simulink model "IEEE9_SG_GFOR_GFOL"  (R2023b)
settings: Solver=ode1  StartTime=0.0  StopTime=sim_config.Tsim  RelTol=1e-3
undefined symbols (not defined in the file): sim_config
libraries: myLibrary x24, spsThreePhaseVIMeasurementLib x12, spsPower3phInstantaneousLib x6, spspowerguiLib x1
settings Model: Creator=Josep  LastModifiedBy=Josep

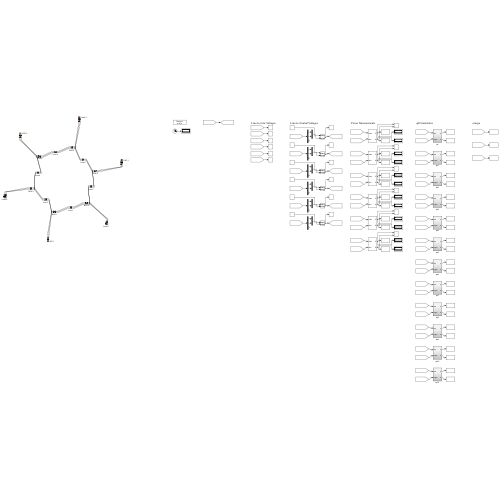
[thumbnail: Simulink's stored preview of the top-level diagram]
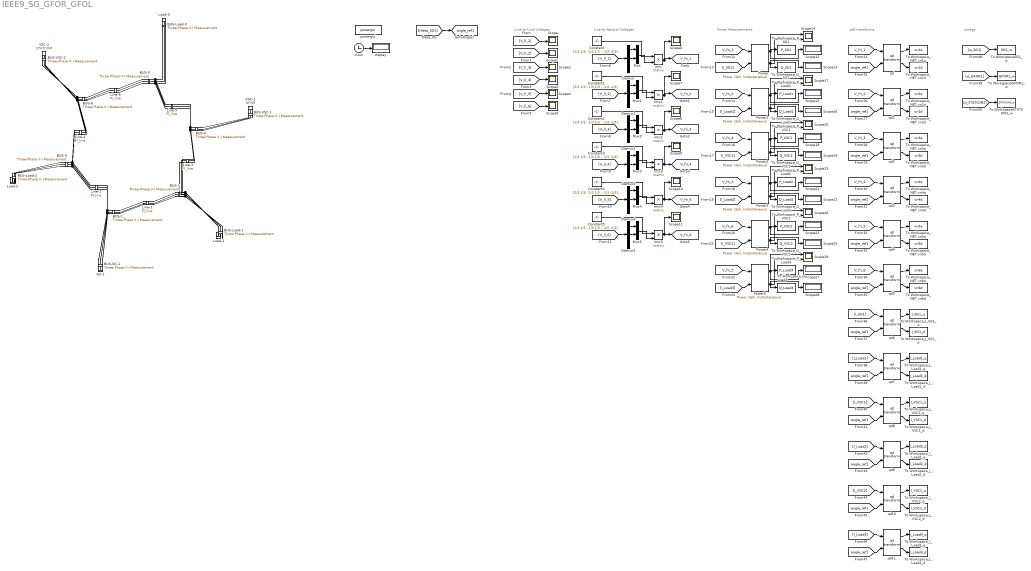
== system IEEE9_SG_GFOR_GFOL ==
  note: Line-to-Line Voltages
  note: Line-to-Neutral Voltages
  note: Power Measurements
  note: qd0 transforms
  note: omega
  BUS-1 : spsThreePhaseVIMeasurementLib/Three-Phase V-I Measurement  VoltageMeasurement=phase-to-phase  SetLabelV=on  LabelV=V_ll_1  Vpu=off  VpuLL=off  CurrentMeasurement=yes  SetLabelI=on  LabelI=I_1  Ipu=off  Pbase=100e6  Vbase=500e3  OutputType=Complex  PhasorSimulation=off  PSBequivalent=0
  BUS-2 : spsThreePhaseVIMeasurementLib/Three-Phase V-I Measurement  VoltageMeasurement=phase-to-phase  SetLabelV=on  LabelV=V_ll_2  Vpu=off  VpuLL=off  CurrentMeasurement=yes  SetLabelI=on  LabelI=I_2  Ipu=off  Pbase=100e6  Vbase=500e3  OutputType=Complex  PhasorSimulation=off  PSBequivalent=0
  BUS-3 : spsThreePhaseVIMeasurementLib/Three-Phase V-I Measurement  VoltageMeasurement=phase-to-phase  SetLabelV=on  LabelV=V_ll_3  Vpu=off  VpuLL=off  CurrentMeasurement=yes  SetLabelI=on  LabelI=I_3  Ipu=off  Pbase=100e6  Vbase=500e3  OutputType=Complex  PhasorSimulation=off  PSBequivalent=0
  BUS-4 : spsThreePhaseVIMeasurementLib/Three-Phase V-I Measurement  VoltageMeasurement=phase-to-phase  SetLabelV=on  LabelV=V_ll_4  Vpu=off  VpuLL=off  CurrentMeasurement=yes  SetLabelI=on  LabelI=I_4  Ipu=off  Pbase=100e6  Vbase=500e3  OutputType=Complex  PhasorSimulation=off  PSBequivalent=0
  BUS-5 : spsThreePhaseVIMeasurementLib/Three-Phase V-I Measurement  VoltageMeasurement=phase-to-phase  SetLabelV=on  LabelV=V_ll_5  Vpu=off  VpuLL=off  CurrentMeasurement=yes  SetLabelI=on  LabelI=I_5  Ipu=off  Pbase=100e6  Vbase=500e3  OutputType=Complex  PhasorSimulation=off  PSBequivalent=0
  BUS-6 : spsThreePhaseVIMeasurementLib/Three-Phase V-I Measurement  VoltageMeasurement=phase-to-phase  SetLabelV=on  LabelV=V_ll_6  Vpu=off  VpuLL=off  CurrentMeasurement=yes  SetLabelI=on  LabelI=I_6  Ipu=off  Pbase=100e6  Vbase=500e3  OutputType=Complex  PhasorSimulation=off  PSBequivalent=0
  BUS-Load-1 : spsThreePhaseVIMeasurementLib/Three-Phase V-I Measurement  VoltageMeasurement=phase-to-phase  SetLabelV=on  LabelV=V_Load_1  Vpu=off  VpuLL=off  CurrentMeasurement=yes  SetLabelI=on  LabelI=I_Load1  Ipu=off  Pbase=100e6  Vbase=500e3  OutputType=Complex  PhasorSimulation=off  PSBequivalent=0
  BUS-Load-2 : spsThreePhaseVIMeasurementLib/Three-Phase V-I Measurement  VoltageMeasurement=phase-to-phase  SetLabelV=on  LabelV=V_Load_2  Vpu=off  VpuLL=off  CurrentMeasurement=yes  SetLabelI=on  LabelI=I_Load2  Ipu=off  Pbase=100e6  Vbase=500e3  OutputType=Complex  PhasorSimulation=off  PSBequivalent=0
  BUS-Load-3 : spsThreePhaseVIMeasurementLib/Three-Phase V-I Measurement  VoltageMeasurement=phase-to-phase  SetLabelV=on  LabelV=V_Load_3  Vpu=off  VpuLL=off  CurrentMeasurement=yes  SetLabelI=on  LabelI=I_Load3  Ipu=off  Pbase=100e6  Vbase=500e3  OutputType=Complex  PhasorSimulation=off  PSBequivalent=0
  BUS-SG-1 : spsThreePhaseVIMeasurementLib/Three-Phase V-I Measurement  VoltageMeasurement=phase-to-phase  SetLabelV=on  LabelV=V_SG_1  Vpu=off  VpuLL=off  CurrentMeasurement=yes  SetLabelI=on  LabelI=I_SG1  Ipu=off  Pbase=100e6  Vbase=500e3  OutputType=Complex  PhasorSimulation=off  PSBequivalent=0
  BUS-VSC-1 : spsThreePhaseVIMeasurementLib/Three-Phase V-I Measurement  VoltageMeasurement=phase-to-phase  SetLabelV=on  LabelV=V_VSC_1  Vpu=off  VpuLL=off  CurrentMeasurement=yes  SetLabelI=on  LabelI=I_VSC1  Ipu=off  Pbase=100e6  Vbase=500e3  OutputType=Complex  PhasorSimulation=off  PSBequivalent=0
  BUS-VSC-2 : spsThreePhaseVIMeasurementLib/Three-Phase V-I Measurement  VoltageMeasurement=phase-to-phase  SetLabelV=on  LabelV=V_VSC_2  Vpu=off  VpuLL=off  CurrentMeasurement=yes  SetLabelI=on  LabelI=I_VSC2  Ipu=off  Pbase=100e6  Vbase=500e3  OutputType=Complex  PhasorSimulation=off  PSBequivalent=0
  Constant{,1..5} (6 alike) : Constant  Value=[2/3 1/3; -1/3 1/3 ; -1/3 -2/3]
  Demux{,1..5} (6 alike) : Demux  Outputs=3
  Line-1 : myLibrary/PI_line  T_line_global=T_NET  initLine_global=init_line  num=1  set_C0=ones(1,6)  set_iL0=0
  Line-2 : myLibrary/PI_line  T_line_global=T_NET  initLine_global=init_line  num=2  set_C0=ones(1,6)  set_iL0=0
  Line-3 : myLibrary/PI_line  T_line_global=T_NET  initLine_global=init_line  num=3  set_C0=ones(1,6)  set_iL0=0
  Line-4 : myLibrary/PI_line  T_line_global=T_NET  initLine_global=init_line  num=4  set_C0=ones(1,6)  set_iL0=0
  Line-5 : myLibrary/PI_line  T_line_global=T_NET  initLine_global=init_line  num=5  set_C0=ones(1,6)  set_iL0=0
  Line-6 : myLibrary/PI_line  T_line_global=T_NET  initLine_global=init_line  num=6  set_C0=ones(1,6)  set_iL0=0
  Load-1 : myLibrary/Load  T_load_global=T_load  initLoad_global=init_load  num=1
  Load-2 : myLibrary/Load  T_load_global=T_load  initLoad_global=init_load  num=2
  Load-3 : myLibrary/Load  T_load_global=T_load  initLoad_global=init_load  num=3
  Mux{,1..5} (6 alike) : Mux  Inputs=2
  Power{,1..5} (6 alike) : spsPower3phInstantaneousLib/Power (3ph, Instantaneous)
  SG-1 : myLibrary/SG  num=1  init_SG_global=init_SG  initMachineBlocks=initMachineBlocks  T_SG_global=T_SG
  Scope{,1..11} (12 alike) : Scope
  Scope{12..13,15..16,18..19,21..22,24..25,27..28} (12 alike) : Display
  Scope{14,17,20,23,26,29} (6 alike) : Scope  NumInputPorts=2
  To WorkspaceGFOR1_w : ToWorkspace  VariableName=GFOR1_w  SampleTime=sim_config.Tsample
  To WorkspaceSG1_w : ToWorkspace  VariableName=SG1_w  SampleTime=sim_config.Tsample
  To WorkspaceSTATCOM2_w : ToWorkspace  VariableName=STATCOM2_w  SampleTime=sim_config.Tsample
  To Workspace_I_Load1_d : ToWorkspace  VariableName=I_Load1_d  SampleTime=sim_config.Tsample
  To Workspace_I_Load1_q : ToWorkspace  VariableName=I_Load1_q  SampleTime=sim_config.Tsample
  To Workspace_I_Load2_d : ToWorkspace  VariableName=I_Load2_d  SampleTime=sim_config.Tsample
  To Workspace_I_Load2_q : ToWorkspace  VariableName=I_Load2_q  SampleTime=sim_config.Tsample
  To Workspace_I_Load3_d : ToWorkspace  VariableName=I_Load3_d  SampleTime=sim_config.Tsample
  To Workspace_I_Load3_q : ToWorkspace  VariableName=I_Load3_q  SampleTime=sim_config.Tsample
  To Workspace_I_SG1_d : ToWorkspace  VariableName=I_SG1_d  SampleTime=sim_config.Tsample
  To Workspace_I_SG1_q : ToWorkspace  VariableName=I_SG1_q  SampleTime=sim_config.Tsample
  To Workspace_I_VSC1_d : ToWorkspace  VariableName=I_VSC1_d  SampleTime=sim_config.Tsample
  To Workspace_I_VSC1_q : ToWorkspace  VariableName=I_VSC1_q  SampleTime=sim_config.Tsample
  To Workspace_I_VSC2_d : ToWorkspace  VariableName=I_VSC2_d  SampleTime=sim_config.Tsample
  To Workspace_I_VSC2_q : ToWorkspace  VariableName=I_VSC2_q  SampleTime=sim_config.Tsample
  To Workspace_NET.vn1d : ToWorkspace  VariableName=vn1d  SampleTime=sim_config.Tsample
  To Workspace_NET.vn1q : ToWorkspace  VariableName=vn1q  SampleTime=sim_config.Tsample
  To Workspace_NET.vn2d : ToWorkspace  VariableName=vn2d  SampleTime=sim_config.Tsample
  To Workspace_NET.vn2q : ToWorkspace  VariableName=vn2q  SampleTime=sim_config.Tsample
  To Workspace_NET.vn3d : ToWorkspace  VariableName=vn3d  SampleTime=sim_config.Tsample
  To Workspace_NET.vn3q : ToWorkspace  VariableName=vn3q  SampleTime=sim_config.Tsample
  To Workspace_NET.vn4d : ToWorkspace  VariableName=vn4d  SampleTime=sim_config.Tsample
  To Workspace_NET.vn4q : ToWorkspace  VariableName=vn4q  SampleTime=sim_config.Tsample
  To Workspace_NET.vn5d : ToWorkspace  VariableName=vn5d  SampleTime=sim_config.Tsample
  To Workspace_NET.vn5q : ToWorkspace  VariableName=vn5q  SampleTime=sim_config.Tsample
  To Workspace_NET.vn6d : ToWorkspace  VariableName=vn6d  SampleTime=sim_config.Tsample
  To Workspace_NET.vn6q : ToWorkspace  VariableName=vn6q  SampleTime=sim_config.Tsample
  To Workspace_P_Load1 : ToWorkspace  VariableName=P_Load1  SampleTime=sim_config.Tsample
  To Workspace_P_Load2 : ToWorkspace  VariableName=P_Load2  SampleTime=sim_config.Tsample
  To Workspace_P_Load3 : ToWorkspace  VariableName=P_Load3  SampleTime=sim_config.Tsample
  To Workspace_P_SG1 : ToWorkspace  VariableName=P_SG1  SampleTime=sim_config.Tsample
  To Workspace_P_VSC1 : ToWorkspace  VariableName=P_VSC1  SampleTime=sim_config.Tsample
  To Workspace_P_VSC2 : ToWorkspace  VariableName=P_VSC2  SampleTime=sim_config.Tsample
  To Workspace_Q_Load1 : ToWorkspace  VariableName=Q_Load1  SampleTime=sim_config.Tsample
  To Workspace_Q_Load2 : ToWorkspace  VariableName=Q_Load2  SampleTime=sim_config.Tsample
  To Workspace_Q_Load3 : ToWorkspace  VariableName=Q_Load3  SampleTime=sim_config.Tsample
  To Workspace_Q_SG1 : ToWorkspace  VariableName=Q_SG1  SampleTime=sim_config.Tsample
  To Workspace_Q_VSC1 : ToWorkspace  VariableName=Q_VSC1  SampleTime=sim_config.Tsample
  To Workspace_Q_VSC2 : ToWorkspace  VariableName=Q_VSC2  SampleTime=sim_config.Tsample
  VSC-1 : myLibrary/GFOR  T_VSC_global=T_VSC  initVSC_global=init_VSC  num=1
  VSC-2 : myLibrary/STATCOM  T_VSC_global=T_VSC  initVSC_global=init_VSC  num=2
  clock : Clock
  display : Display
  mtx{,1..5} (6 alike) : Product  Multiplication=Matrix(*)
  powergui : spspowerguiLib/powergui  Priority=1  SimulationMode=Discrete  SampleTime=sim_config.Ts  frequency=60  Iterations=50  frequencyindice=60  Pbase=100e6  ErrMax=1e-4  UnitsV=kV  UnitsW=MW  buscounter=0  FunctionMessages=off  echomessages=off  EnableUseOfTLC=off  CurrentSourceSwitches=off  DisableSnubberDevices=off  DisableRonSwitches=off  DisableVfSwitches=off  DisplayEquations=off  AutomaticDiscreteSolvers=off  SolverType=Tustin/Backward Euler (TBE)  Interpol=off  ExternalGateDelay=off  methode=off  Ts=100  x0status=blocks  SPID=on  SwTol=0  HookPort=off  NonlinearTolerance=1e-4  nMaxIteration=100  ContinueOnMaxIteration=off  RestoreLinks=warning  ResistiveCurrentMeasurement=off  Frange=[0:2:500]  Ylog=off  Xlog=on  ShowGrid=off  save=off  variable=ZData  structure=0  ZoomFFT=off  StartTime=0.0  cycles=1  DisplayStyle=1  fundamental=60  FreqAxis=off  MaxFrequency=1000  frequencyindicesteady=1  RmsSteady=1  display=off
  qd{,1..11} (12 alike) : myLibrary/qd transform  SystemSampleTime=-1  VariantActivationTime=update diagram  AllowFlexibleInterface=on  Latency=0  AutoFrameSizeCalculation=off
  tag scope: V_fn_1=global, V_fn_2=global, V_fn_3=global, V_fn_4=global, V_fn_5=global, V_fn_6=global, angle_ref1=global
  wires:
  clock/1 -> display/1
  [theta_SG1] -> [angle_ref1]
  [V_ll_1] -> Scope/1
  [V_ll_2] -> Scope1/1
  [V_ll_3] -> Scope2/1
  [V_ll_4] -> Scope3/1
  [V_ll_5] -> Scope4/1
  [V_ll_6] -> Scope5/1
  [V_ll_1] -> Demux/1
  Demux/1 -> Mux/1
  Demux/2 -> Mux/2
  Mux/1 -> mtx/2
  Constant/1 -> mtx/1
  mtx/1 -> [V_fn_1], Scope6/1
  [V_ll_2] -> Demux1/1
  Demux1/1 -> Mux1/1
  Demux1/2 -> Mux1/2
  Mux1/1 -> mtx1/2
  Constant1/1 -> mtx1/1
  mtx1/1 -> [V_fn_2], Scope7/1
  [V_ll_3] -> Demux2/1
  Demux2/1 -> Mux2/1
  Demux2/2 -> Mux2/2
  Mux2/1 -> mtx2/2
  Constant2/1 -> mtx2/1
  mtx2/1 -> [V_fn_3], Scope8/1
  [V_ll_4] -> Demux3/1
  Demux3/1 -> Mux3/1
  Demux3/2 -> Mux3/2
  Mux3/1 -> mtx3/2
  Constant3/1 -> mtx3/1
  mtx3/1 -> [V_fn_4], Scope9/1
  [V_ll_5] -> Demux4/1
  Demux4/1 -> Mux4/1
  Demux4/2 -> Mux4/2
  Mux4/1 -> mtx4/2
  Constant4/1 -> mtx4/1
  mtx4/1 -> [V_fn_5], Scope10/1
  [V_ll_6] -> Demux5/1
  Demux5/1 -> Mux5/1
  Demux5/2 -> Mux5/2
  Mux5/1 -> mtx5/2
  Constant5/1 -> mtx5/1
  mtx5/1 -> [V_fn_6], Scope11/1
  [V_fn_1] -> Power/1
  [I_SG1] -> Power/2
  Power/1 -> To Workspace_P_SG1/1, Scope12/1, Scope14/1
  Power/2 -> To Workspace_Q_SG1/1, Scope13/1, Scope14/2
  [V_fn_2] -> Power1/1
  [I_Load1] -> Power1/2
  Power1/1 -> To Workspace_P_Load1/1, Scope15/1, Scope17/1
  Power1/2 -> To Workspace_Q_Load1/1, Scope16/1, Scope17/2
  [V_fn_4] -> Power2/1
  [I_VSC1] -> Power2/2
  Power2/1 -> To Workspace_P_VSC1/1, Scope18/1, Scope20/1
  Power2/2 -> To Workspace_Q_VSC1/1, Scope19/1, Scope20/2
  [V_fn_3] -> Power3/1
  [I_Load2] -> Power3/2
  Power3/1 -> To Workspace_P_Load2/1, Scope21/1, Scope23/1
  Power3/2 -> To Workspace_Q_Load2/1, Scope22/1, Scope23/2
  [V_fn_6] -> Power4/1
  [I_VSC2] -> Power4/2
  Power4/1 -> To Workspace_P_VSC2/1, Scope24/1, Scope26/1
  Power4/2 -> To Workspace_Q_VSC2/1, Scope25/1, Scope26/2
  [V_fn_5] -> Power5/1
  [I_Load3] -> Power5/2
  Power5/1 -> To Workspace_P_Load3/1, Scope27/1, Scope29/1
  Power5/2 -> To Workspace_Q_Load3/1, Scope28/1, Scope29/2
  [V_fn_1] -> qd/1
  [angle_ref1] -> qd/2
  qd/1 -> To Workspace_NET.vn1q/1
  qd/2 -> To Workspace_NET.vn1d/1
  [V_fn_2] -> qd1/1
  [angle_ref1] -> qd1/2
  qd1/1 -> To Workspace_NET.vn2q/1
  qd1/2 -> To Workspace_NET.vn2d/1
  [V_fn_3] -> qd2/1
  [angle_ref1] -> qd2/2
  qd2/1 -> To Workspace_NET.vn3q/1
  qd2/2 -> To Workspace_NET.vn3d/1
  [V_fn_4] -> qd3/1
  [angle_ref1] -> qd3/2
  qd3/1 -> To Workspace_NET.vn4q/1
  qd3/2 -> To Workspace_NET.vn4d/1
  [V_fn_5] -> qd4/1
  [angle_ref1] -> qd4/2
  qd4/1 -> To Workspace_NET.vn5q/1
  qd4/2 -> To Workspace_NET.vn5d/1
  [V_fn_6] -> qd5/1
  [angle_ref1] -> qd5/2
  qd5/1 -> To Workspace_NET.vn6q/1
  qd5/2 -> To Workspace_NET.vn6d/1
  [I_SG1] -> qd6/1
  [angle_ref1] -> qd6/2
  qd6/1 -> To Workspace_I_SG1_q/1
  qd6/2 -> To Workspace_I_SG1_d/1
  [I_Load1] -> qd7/1
  [angle_ref1] -> qd7/2
  qd7/1 -> To Workspace_I_Load1_q/1
  qd7/2 -> To Workspace_I_Load1_d/1
  [I_VSC1] -> qd8/1
  [angle_ref1] -> qd8/2
  qd8/1 -> To Workspace_I_VSC1_q/1
  qd8/2 -> To Workspace_I_VSC1_d/1
  [I_Load2] -> qd9/1
  [angle_ref1] -> qd9/2
  qd9/1 -> To Workspace_I_Load2_q/1
  qd9/2 -> To Workspace_I_Load2_d/1
  [I_VSC2] -> qd10/1
  [angle_ref1] -> qd10/2
  qd10/1 -> To Workspace_I_VSC2_q/1
  qd10/2 -> To Workspace_I_VSC2_d/1
  [I_Load3] -> qd11/1
  [angle_ref1] -> qd11/2
  qd11/1 -> To Workspace_I_Load3_q/1
  qd11/2 -> To Workspace_I_Load3_d/1
  [w_SG1] -> To WorkspaceSG1_w/1
  [w_GFOR1] -> To WorkspaceGFOR1_w/1
  [w_STATCOM2] -> To WorkspaceSTATCOM2_w/1
  connections:
  BUS-SG-1/RConn1 -- BUS-1/LConn1 -- Line-2/LConn1
  BUS-SG-1/RConn2 -- BUS-1/LConn2 -- Line-2/LConn2
  BUS-SG-1/RConn3 -- BUS-1/LConn3 -- Line-2/LConn3
  BUS-SG-1/LConn1 -- SG-1/RConn1
  BUS-SG-1/LConn2 -- SG-1/RConn2
  BUS-SG-1/LConn3 -- SG-1/RConn3
  BUS-1/RConn1 -- Line-1/LConn1
  BUS-1/RConn2 -- Line-1/LConn2
  BUS-1/RConn3 -- Line-1/LConn3
  Line-1/RConn1 -- BUS-2/LConn1
  Line-1/RConn2 -- BUS-2/LConn2
  Line-1/RConn3 -- BUS-2/LConn3
  BUS-Load-1/LConn1 -- BUS-2/RConn1 -- Line-3/LConn1
  BUS-Load-1/LConn2 -- BUS-2/RConn2 -- Line-3/LConn2
  BUS-Load-1/LConn3 -- BUS-2/RConn3 -- Line-3/LConn3
  BUS-Load-1/RConn1 -- Load-1/LConn1
  BUS-Load-1/RConn2 -- Load-1/LConn2
  BUS-Load-1/RConn3 -- Load-1/LConn3
  BUS-4/LConn1 -- Line-3/RConn1 -- Line-5/LConn1
  BUS-4/LConn2 -- Line-3/RConn2 -- Line-5/LConn2
  BUS-4/LConn3 -- Line-3/RConn3 -- Line-5/LConn3
  BUS-4/RConn1 -- BUS-VSC-1/RConn1
  BUS-4/RConn2 -- BUS-VSC-1/RConn2
  BUS-4/RConn3 -- BUS-VSC-1/RConn3
  BUS-VSC-1/LConn1 -- VSC-1/RConn1
  BUS-VSC-1/LConn2 -- VSC-1/RConn2
  BUS-VSC-1/LConn3 -- VSC-1/RConn3
  BUS-5/RConn1 -- Line-5/RConn1 -- BUS-Load-3/LConn1
  BUS-5/RConn2 -- Line-5/RConn2 -- BUS-Load-3/LConn2
  BUS-5/RConn3 -- Line-5/RConn3 -- BUS-Load-3/LConn3
  BUS-Load-3/RConn1 -- Load-3/LConn1
  BUS-Load-3/RConn2 -- Load-3/LConn2
  BUS-Load-3/RConn3 -- Load-3/LConn3
  BUS-5/LConn1 -- Line-6/LConn1
  BUS-5/LConn2 -- Line-6/LConn2
  BUS-5/LConn3 -- Line-6/LConn3
  Line-6/RConn1 -- BUS-6/RConn1
  Line-6/RConn2 -- BUS-6/RConn2
  Line-6/RConn3 -- BUS-6/RConn3
  BUS-VSC-2/RConn1 -- BUS-6/LConn1 -- Line-4/RConn1
  BUS-VSC-2/RConn2 -- BUS-6/LConn2 -- Line-4/RConn2
  BUS-VSC-2/RConn3 -- BUS-6/LConn3 -- Line-4/RConn3
  BUS-VSC-2/LConn1 -- VSC-2/RConn1
  BUS-VSC-2/LConn2 -- VSC-2/RConn2
  BUS-VSC-2/LConn3 -- VSC-2/RConn3
  Line-4/LConn1 -- BUS-3/RConn1 -- Line-2/RConn1
  Line-4/LConn2 -- BUS-3/RConn2 -- Line-2/RConn2
  Line-4/LConn3 -- BUS-3/RConn3 -- Line-2/RConn3
  BUS-3/LConn1 -- BUS-Load-2/LConn1
  BUS-3/LConn2 -- BUS-Load-2/LConn2
  BUS-3/LConn3 -- BUS-Load-2/LConn3
  BUS-Load-2/RConn1 -- Load-2/LConn1
  BUS-Load-2/RConn2 -- Load-2/LConn2
  BUS-Load-2/RConn3 -- Load-2/LConn3
